simulink model "balancing_sim_model_induced_voltage"  (R2016a)
settings: Solver=ode4  StartTime=0.0  StopTime=Tfinal  FixedStep=Ts  RelTol=1e-3
values from neighbouring files (symbols this model uses):
  Cdc = 15e-6    (= 1.5e-05)    [balancing_sim_parameters.m]    (also in rectifier_sim_parameters.m; sixthharmonicstudies_another_sim_param.m)
  delta1 = acos(Ef1_avg/Vt1)    [balancing_sim_parameters.m]
  delta2 = acos(Ef2_avg/Vt2)    [balancing_sim_parameters.m]
  Ef1A = 80    [balancing_sim_parameters.m]
  Ef1A_ph = 0    [balancing_sim_parameters.m]
  Ef1B = Ef1A    (= 80)    [balancing_sim_parameters.m]
  Ef1B_ph = Ef1A_ph - 120    (= -120)    [balancing_sim_parameters.m]
  Ef1C = Ef1A    (= 80)    [balancing_sim_parameters.m]
  Ef1C_ph = Ef1A_ph + 120    (= 120)    [balancing_sim_parameters.m]
  Ef2A = 90    [balancing_sim_parameters.m]
  Ef2A_ph = 0    [balancing_sim_parameters.m]
  Ef2B = Ef2A    (= 90)    [balancing_sim_parameters.m]
  Ef2B_ph = Ef2A_ph - 120    (= -120)    [balancing_sim_parameters.m]
  Ef2C = Ef2A    (= 90)    [balancing_sim_parameters.m]
  Ef2C_ph = Ef2A_ph + 120    (= 120)    [balancing_sim_parameters.m]
  fout = 75    [balancing_sim_parameters.m]    (also in balancing_voltage_calc.m = 50; rectifier_sim_parameters.m = 50; sixthharmonicstudies_another_sim_param.m = 150)
  Ls = 10e-3    (= 0.01)    [balancing_sim_parameters.m]
  ma1 = 0.9    [balancing_sim_parameters.m]    (also in balancing_voltage_calc.m; rectifier_sim_parameters.m; sixthharmonicstudies_another_sim_param.m)
  ma2 = 0.9    [balancing_sim_parameters.m]    (also in balancing_voltage_calc.m)
  phase = [0 90 0 90]    [balancing_sim_parameters.m]    (also in rectifier_sim_parameters.m; sixthharmonicstudies_another_sim_param.m)
  Rin = 70    [balancing_sim_parameters.m]    (also in rectifier_sim_parameters.m = 10; sixthharmonicstudies_another_sim_param.m = 10)
  Ripth = 0.04    [balancing_sim_parameters.m]    (also in rectifier_sim_parameters.m = 0.18; sixthharmonicstudies_another_sim_param.m = 0.18)
  Rs = 1e-3    (= 0.001)    [balancing_sim_parameters.m]
  Ts = 1e-7    (= 1e-07)    [balancing_sim_parameters.m]    (also in rectifier_sim_parameters.m = 1e-06; sixthharmonicstudies_another_sim_param.m = 1e-06)
  Vin = Vdc + Rin*(Pout/Vdc)+3    (= 1061.51851852)    [balancing_sim_parameters.m]    (also in rectifier_sim_parameters.m = 366.296296296; sixthharmonicstudies_another_sim_param.m = 344.814814815)
  wout = 2*pi*fout    (= 471.238898038)    [balancing_sim_parameters.m]    (also in rectifier_sim_parameters.m = 314.159265359; sixthharmonicstudies_another_sim_param.m = 942.477796077)
undefined symbols (not defined in the file or in its folder): Lload, Rload
libraries: powerlib x47, powerlib_meascontrol x29, simulink x8
settings Model: SimulationMode=accelerator  Creator=ugurm  LastModifiedBy=mesutto
settings DataIOCC: LimitDataPoints=on  SaveFormat=Array
settings DebuggingCC: UnderspecifiedInitializationDetection=Classic  MergeDetectMultiDrivingBlocksExec=none  SolverPrmCheckMsg=warning  StateNameClashWarn=warning
settings HardwareCC: ProdBitPerPointer=32  ProdLargestAtomicFloat=None  ProdIntDivRoundTo=Undefined  ProdEndianess=Unspecified  ProdWordSize=32  ProdHWDeviceType=32-bit Generic
settings ModelReferenceCC: PropagateSignalLabelsOutOfModel=off
settings ConfigComp: CovModelRefEnable=Off

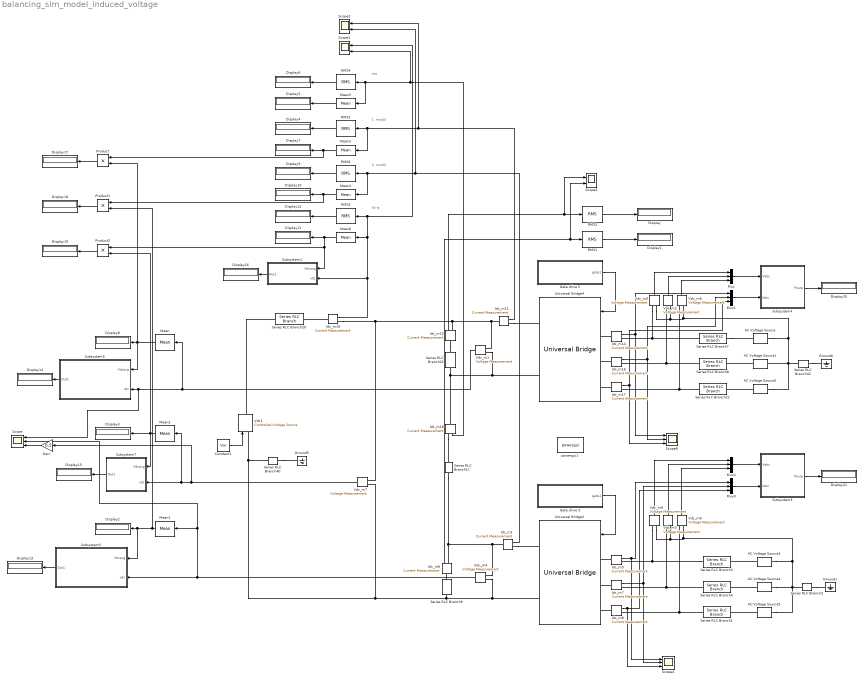
== system balancing_sim_model_induced_voltage ==
  note: 1. modül
  note: 2. modül
  note: ara
  note: Giriş
  AC Voltage Source : powerlib/Electrical Sources/AC Voltage Source  Amplitude=Ef1A*sqrt(2)  Phase=Ef1A_ph  Frequency=fout  SampleTime=0  Measurements=None  BusType=swing  Pref=10e3  Qref=0  Qmin=-inf  Qmax=+inf
  AC Voltage Source1 : powerlib/Electrical Sources/AC Voltage Source  Amplitude=Ef1B*sqrt(2)  Phase=Ef1B_ph  Frequency=fout  SampleTime=0  Measurements=None  BusType=swing  Pref=10e3  Qref=0  Qmin=-inf  Qmax=+inf
  AC Voltage Source2 : powerlib/Electrical Sources/AC Voltage Source  Amplitude=Ef1C*sqrt(2)  Phase=Ef1C_ph  Frequency=fout  SampleTime=0  Measurements=None  BusType=swing  Pref=10e3  Qref=0  Qmin=-inf  Qmax=+inf
  AC Voltage Source3 : powerlib/Electrical Sources/AC Voltage Source  Amplitude=Ef2A*sqrt(2)  Phase=Ef2A_ph  Frequency=fout  SampleTime=0  Measurements=None  BusType=swing  Pref=10e3  Qref=0  Qmin=-inf  Qmax=+inf
  AC Voltage Source4 : powerlib/Electrical Sources/AC Voltage Source  Amplitude=Ef2B*sqrt(2)  Phase=Ef2B_ph  Frequency=fout  SampleTime=0  Measurements=None  BusType=swing  Pref=10e3  Qref=0  Qmin=-inf  Qmax=+inf
  AC Voltage Source5 : powerlib/Electrical Sources/AC Voltage Source  Amplitude=Ef2C*sqrt(2)  Phase=Ef2C_ph  Frequency=fout  SampleTime=0  Measurements=None  BusType=swing  Pref=10e3  Qref=0  Qmin=-inf  Qmax=+inf
  Constant1 : Constant  Value=Vin
  Display{,1..21} (22 alike) : Display
  Gain : Gain  Gain=0.5
  Gate drive 3 : Subsystem
  Gate drive 5 : Subsystem
  Ground1 : powerlib/Elements/Ground  LConnTagsString=a
  Ground5 : powerlib/Elements/Ground  LConnTagsString=a
  Ground6 : powerlib/Elements/Ground  LConnTagsString=a
  Idc_m{1,5..8,11,14..19} (12 alike) : powerlib/Measurements/Current Measurement  PhasorSimulation=off  OutputType=Complex  PSBequivalent=0
  Mean{,1..6} (7 alike) : powerlib_meascontrol/Measurements/Mean  Freq=fout  Vinit=0  Ts=0
  Mux{,1..3} (4 alike) : Mux  Inputs=3
  Product : Product
  Product1 : Product
  Product2 : Product
  RMS{1..6} (6 alike) : powerlib_meascontrol/Measurements/RMS  TrueRMS=on  Freq=fout  RMSInit=0  Ts=0
  Scope : Scope  NumInputPorts=3
  Scope1 : Scope  NumInputPorts=2
  Scope2 : Scope  NumInputPorts=2
  Scope3 : Scope  NumInputPorts=2
  Scope4 : Scope  NumInputPorts=3
  Scope8 : Scope  NumInputPorts=3
  Series RLC Branch{1,3..4,7..8,22} (6 alike) : powerlib/Elements/Series RLC Branch  LConnTagsString=__new0  RConnTagsString=__new0  BranchType=RL  Resistance=Rs  Inductance=Ls  SetiL0=off  InitialCurrent=0  Capacitance=1e-6  Setx0=off  InitialVoltage=0  Measurements=None
  Series RLC Branch17 : powerlib/Elements/Series RLC Branch  LConnTagsString=__new0  RConnTagsString=__new0  BranchType=R  Resistance=1e-6  Inductance=Lload  SetiL0=off  InitialCurrent=0  Capacitance=1e-6  Setx0=off  InitialVoltage=0  Measurements=None
  Series RLC Branch2 : powerlib/Elements/Series RLC Branch  LConnTagsString=__new0  RConnTagsString=__new0  BranchType=R  Resistance=1e12  Inductance=Lload  SetiL0=off  InitialCurrent=0  Capacitance=1e-6  Setx0=off  InitialVoltage=0  Measurements=None
  Series RLC Branch20 : powerlib/Elements/Series RLC Branch  LConnTagsString=__new0  RConnTagsString=__new0  BranchType=R  Resistance=Rin  Inductance=1e-3  SetiL0=off  InitialCurrent=0  Capacitance=1e-6  Setx0=off  InitialVoltage=0  Measurements=None
  Series RLC Branch21 : powerlib/Elements/Series RLC Branch  LConnTagsString=__new0  RConnTagsString=__new0  BranchType=C  Resistance=Rload  Inductance=Lload  SetiL0=off  InitialCurrent=0  Capacitance=Cdc  Setx0=off  InitialVoltage=0  Measurements=None
  Series RLC Branch40 : powerlib/Elements/Series RLC Branch  LConnTagsString=__new0  RConnTagsString=__new0  BranchType=R  Resistance=1e12  Inductance=Lload  SetiL0=off  InitialCurrent=0  Capacitance=1e-6  Setx0=off  InitialVoltage=0  Measurements=None
  Series RLC Branch42 : powerlib/Elements/Series RLC Branch  LConnTagsString=__new0  RConnTagsString=__new0  BranchType=R  Resistance=1e12  Inductance=Lload  SetiL0=off  InitialCurrent=0  Capacitance=1e-6  Setx0=off  InitialVoltage=0  Measurements=None
  Series RLC Branch9 : powerlib/Elements/Series RLC Branch  LConnTagsString=__new0  RConnTagsString=__new0  BranchType=C  Resistance=Rload  Inductance=Lload  SetiL0=off  InitialCurrent=0  Capacitance=Cdc  Setx0=off  InitialVoltage=0  Measurements=None
  Subsystem1 : Subsystem
  Subsystem2 : Subsystem
  Subsystem3 : Subsystem
  Subsystem4 : Subsystem
  Subsystem5 : Subsystem
  Subsystem7 : Subsystem
  Universal Bridge3 : powerlib/Power Electronics/Universal Bridge  Arms=3  SnubberResistance=1e5  SnubberCapacitance=inf  Device=IGBT / Diodes  Ron=1e-6  Lon=0  ForwardVoltages="[  0  0  ]"  ForwardVoltage=0  GTOparameters=[ 10e-6 , 20e-6 ]  IGBTparameters=[0,0]  Measurements=None  Measurements_2=None  converterType=Rectifier
  Universal Bridge4 : powerlib/Power Electronics/Universal Bridge  Arms=3  SnubberResistance=1e5  SnubberCapacitance=inf  Device=IGBT / Diodes  Ron=1e-6  Lon=0  ForwardVoltages="[  0  0  ]"  ForwardVoltage=0  GTOparameters=[ 10e-6 , 20e-6 ]  IGBTparameters=[0,0]  Measurements=None  Measurements_2=None  converterType=Rectifier
  Vdc1 : powerlib/Electrical Sources/Controlled Voltage Source  Initialize=off  Source_Type=DC  Amplitude=200  Phase=0  Frequency=0  Measurements=None
  Vdc_m{1..9} (9 alike) : powerlib/Measurements/Voltage Measurement  PhasorSimulation=off  OutputType=Complex  PSBequivalent=0
  powergui1 : powerlib/powergui  Priority=1  SimulationMode=Discrete  SolverType=Tustin  SampleTime=Ts  frequency=60  SPID=off  DisableSnubberDevices=off  DisableRonSwitches=off  DisableVfSwitches=off  SwTol=0  DisplayEquations=off  Interpol=off  ExternalGateDelay=off  methode=off  Ts=0  FunctionMessages=off  echomessages=off  HookPort=off  EnableUseOfTLC=off  x0status=blocks  frequencyindice=0  Pbase=100e6  ErrMax=1e-4  Iterations=50  UnitsV=kV  UnitsW=MW  buscounter=0  RestoreLinks=warning  ResistiveCurrentMeasurement=off  Frange=[0:2:500]  Ylog=off  Xlog=on  ShowGrid=off  save=off  variable=ZData  structure=Vdc  ZoomFFT=off  StartTime=0.04  cycles=5  DisplayStyle=5  fundamental=50  FreqAxis=off  MaxFrequency=30000  frequencyindicesteady=1  RmsSteady=1  display=off
  wires:
  Gate drive 5/1(gate1) -> Universal Bridge4/1
  Idc_m14/1 -> Mux1/1, Scope8/1
  Constant1/1 -> Vdc1/1
  Idc_m15/1 -> RMS3/1, Scope3/1
  Vdc_m1/1 -> Mean/1, Scope/1, Subsystem5/2(vdc)
  Idc_m16/1 -> Mux1/2, Scope8/2
  Idc_m17/1 -> Scope8/3, Mux1/3
  RMS3/1 -> Display/1
  Mean/1 -> Product/2, Subsystem5/1(Vdcavg), Display8/1
  Gate drive 3/1(gate1) -> Universal Bridge3/1
  Mean1/1 -> Product1/2, Subsystem2/1(Vdcavg), Display2/1
  Mean2/1 -> Product2/2, Subsystem7/1(Vdcavg), Display3/1
  Vdc_m7/1 -> Gain/1, Subsystem7/2(vdc), Mean2/1
  RMS2/1 -> Display4/1
  Idc_m11/1 -> RMS2/1, Mean3/1, Scope2/1
  Idc_m18/1 -> Scope1/2, Mean5/1, RMS4/1
  Idc_m19/1 -> Subsystem1/2(vdc), Mean6/1, Scope1/1, RMS5/1
  Idc_m6/1 -> Scope3/2, RMS1/1
  RMS1/1 -> Display1/1
  Mean3/1 -> Product/1, Display7/1
  RMS6/1 -> Display9/1
  Mean4/1 -> Display10/1, Product1/1
  RMS4/1 -> Display6/1
  Mean5/1 -> Display5/1
  RMS5/1 -> Display12/1
  Mean6/1 -> Product2/1, Subsystem1/1(Vdcavg), Display11/1
  Idc_m1/1 -> Mean4/1, RMS6/1, Scope2/2
  Subsystem5/1(Out1) -> Display14/1
  Subsystem2/1(Out1) -> Display13/1
  Subsystem7/1(Out1) -> Display15/1
  Subsystem1/1(Out1) -> Display16/1
  Product/1 -> Display17/1
  Product1/1 -> Display18/1
  Vdc_m4/1 -> Scope/2, Mean1/1, Subsystem2/2(vdc)
  Product2/1 -> Display19/1
  Vdc_m5/1 -> Mux/1
  Vdc_m2/1 -> Mux/2
  Vdc_m6/1 -> Mux/3
  Mux/1 -> Subsystem4/1(Vabc)
  Mux1/1 -> Subsystem4/2(Iabc)
  Vdc_m8/1 -> Mux2/1
  Vdc_m3/1 -> Mux2/2
  Vdc_m9/1 -> Mux2/3
  Mux2/1 -> Subsystem3/1(Vabc)
  Mux3/1 -> Subsystem3/2(Iabc)
  Idc_m5/1 -> Scope4/1, Mux3/1
  Idc_m7/1 -> Scope4/2, Mux3/2
  Idc_m8/1 -> Scope4/3, Mux3/3
  Subsystem4/1(Poutp) -> Display20/1
  Subsystem3/1(Poutp) -> Display21/1
  Gain/1 -> Scope/3
  connections:
  Vdc_m5/LConn1 -- Series RLC Branch7/LConn1 -- Idc_m14/RConn1
  Idc_m18/LConn1 -- Vdc_m1/LConn2 -- Universal Bridge4/RConn2 -- Series RLC Branch21/RConn1
  Series RLC Branch42/RConn1 -- Ground6/LConn1
  Series RLC Branch40/RConn1 -- Ground5/LConn1
  Idc_m14/LConn1 -- Universal Bridge4/LConn1
  Idc_m15/LConn1 -- Series RLC Branch21/LConn1
  Vdc1/RConn1 -- Series RLC Branch20/LConn1
  Idc_m16/LConn1 -- Universal Bridge4/LConn2
  Idc_m17/LConn1 -- Universal Bridge4/LConn3
  Vdc_m6/LConn1 -- Series RLC Branch22/LConn1 -- Idc_m17/RConn1
  Vdc_m2/LConn1 -- Series RLC Branch8/LConn1 -- Idc_m16/RConn1
  Vdc_m8/LConn1 -- Series RLC Branch3/LConn1 -- Idc_m5/RConn1
  Series RLC Branch2/LConn1 -- AC Voltage Source4/LConn1 -- AC Voltage Source5/LConn1 -- AC Voltage Source3/LConn1 -- Vdc_m3/LConn2 -- Vdc_m8/LConn2 -- Vdc_m9/LConn2
  Vdc_m3/LConn1 -- Series RLC Branch4/LConn1 -- Idc_m7/RConn1
  Vdc_m9/LConn1 -- Series RLC Branch1/LConn1 -- Idc_m8/RConn1
  Idc_m8/LConn1 -- Universal Bridge3/LConn3
  Idc_m5/LConn1 -- Universal Bridge3/LConn1
  Idc_m7/LConn1 -- Universal Bridge3/LConn2
  Idc_m6/LConn1 -- Series RLC Branch9/LConn1
  Idc_m15/RConn1 -- Vdc_m1/LConn1 -- Idc_m11/LConn1 -- Vdc_m7/LConn1 -- Idc_m19/RConn1
  Series RLC Branch17/RConn1 -- Vdc_m4/LConn1 -- Idc_m1/LConn1 -- Idc_m6/RConn1
  Idc_m11/RConn1 -- Universal Bridge4/RConn1
  Idc_m18/RConn1 -- Series RLC Branch17/LConn1
  Idc_m19/LConn1 -- Series RLC Branch20/RConn1
  Vdc1/LConn1 -- Vdc_m4/LConn2 -- Universal Bridge3/RConn2 -- Series RLC Branch9/RConn1 -- Vdc_m7/LConn2 -- Series RLC Branch40/LConn1
  Idc_m1/RConn1 -- Universal Bridge3/RConn1
  Vdc_m5/LConn2 -- Series RLC Branch42/LConn1 -- AC Voltage Source2/LConn1 -- AC Voltage Source1/LConn1 -- AC Voltage Source/LConn1 -- Vdc_m6/LConn2 -- Vdc_m2/LConn2
  AC Voltage Source1/RConn1 -- Series RLC Branch8/RConn1
  Series RLC Branch7/RConn1 -- AC Voltage Source/RConn1
  AC Voltage Source2/RConn1 -- Series RLC Branch22/RConn1
  AC Voltage Source4/RConn1 -- Series RLC Branch4/RConn1
  AC Voltage Source3/RConn1 -- Series RLC Branch3/RConn1
  AC Voltage Source5/RConn1 -- Series RLC Branch1/RConn1
  Series RLC Branch2/RConn1 -- Ground1/LConn1

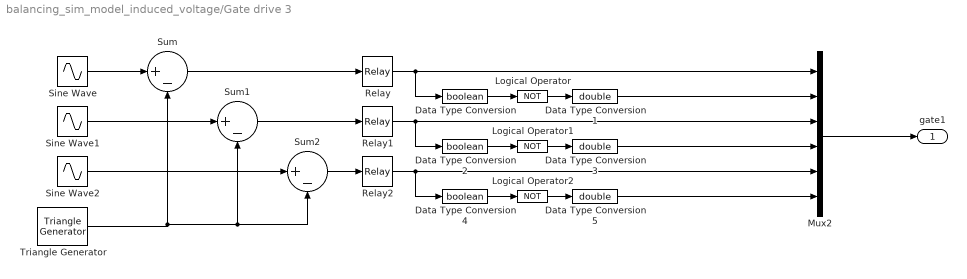
== system balancing_sim_model_induced_voltage/Gate drive 3 ==
  Data Type Conversion : DataTypeConversion  OutDataTypeStr=boolean
  Data Type Conversion1 : DataTypeConversion  OutDataTypeStr=double
  Data Type Conversion2 : DataTypeConversion  OutDataTypeStr=boolean
  Data Type Conversion3 : DataTypeConversion  OutDataTypeStr=double
  Data Type Conversion4 : DataTypeConversion  OutDataTypeStr=boolean
  Data Type Conversion5 : DataTypeConversion  OutDataTypeStr=double
  Logical Operator : Logic  Operator=NOT  AllPortsSameDT=off  OutDataTypeStr=boolean
  Logical Operator1 : Logic  Operator=NOT  AllPortsSameDT=off  OutDataTypeStr=boolean
  Logical Operator2 : Logic  Operator=NOT  AllPortsSameDT=off  OutDataTypeStr=boolean
  Mux2 : Mux  Inputs=6
  Relay : Relay
  Relay1 : Relay
  Relay2 : Relay
  Sine Wave : Sin  Amplitude=ma2  Frequency=wout  Phase=delta2  SampleTime=0
  Sine Wave1 : Sin  Amplitude=ma2  Frequency=wout  Phase=-2*pi/3+delta2  SampleTime=0
  Sine Wave2 : Sin  Amplitude=ma2  Frequency=wout  Phase=2*pi/3+delta2  SampleTime=0
  Sum : Sum  Inputs=|+-
  Sum1 : Sum  Inputs=|+-
  Sum2 : Sum  Inputs=|+-
  Triangle Generator : powerlib_meascontrol/Pulse & Signal Generators/Triangle Generator  Freq=fsw  Phase=phase(3)  Ts=Ts
  gate1 : Outport
  wires:
  Sine Wave/1 -> Sum/1
  Triangle Generator/1 -> Sum1/2, Sum2/2, Sum/2
  Sine Wave1/1 -> Sum1/1
  Sine Wave2/1 -> Sum2/1
  Sum/1 -> Relay/1
  Sum1/1 -> Relay1/1
  Sum2/1 -> Relay2/1
  Data Type Conversion/1 -> Logical Operator/1
  Relay/1 -> Data Type Conversion/1, Mux2/1
  Logical Operator/1 -> Data Type Conversion1/1
  Data Type Conversion1/1 -> Mux2/2
  Data Type Conversion2/1 -> Logical Operator1/1
  Relay1/1 -> Data Type Conversion2/1, Mux2/3
  Logical Operator1/1 -> Data Type Conversion3/1
  Data Type Conversion3/1 -> Mux2/4
  Data Type Conversion4/1 -> Logical Operator2/1
  Relay2/1 -> Data Type Conversion4/1, Mux2/5
  Logical Operator2/1 -> Data Type Conversion5/1
  Data Type Conversion5/1 -> Mux2/6
  Mux2/1 -> gate1/1

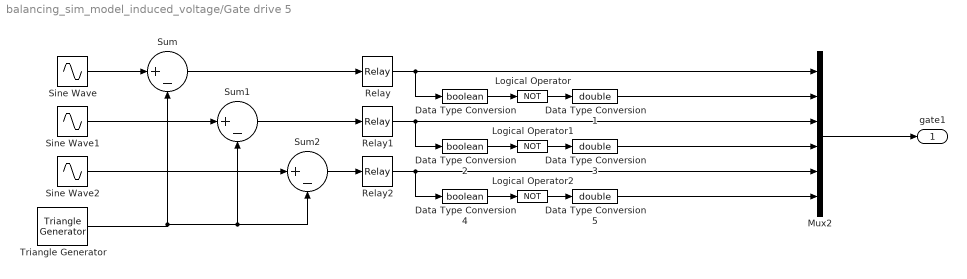
== system balancing_sim_model_induced_voltage/Gate drive 5 ==
  Data Type Conversion : DataTypeConversion  OutDataTypeStr=boolean
  Data Type Conversion1 : DataTypeConversion  OutDataTypeStr=double
  Data Type Conversion2 : DataTypeConversion  OutDataTypeStr=boolean
  Data Type Conversion3 : DataTypeConversion  OutDataTypeStr=double
  Data Type Conversion4 : DataTypeConversion  OutDataTypeStr=boolean
  Data Type Conversion5 : DataTypeConversion  OutDataTypeStr=double
  Logical Operator : Logic  Operator=NOT  AllPortsSameDT=off  OutDataTypeStr=boolean
  Logical Operator1 : Logic  Operator=NOT  AllPortsSameDT=off  OutDataTypeStr=boolean
  Logical Operator2 : Logic  Operator=NOT  AllPortsSameDT=off  OutDataTypeStr=boolean
  Mux2 : Mux  Inputs=6
  Relay : Relay
  Relay1 : Relay
  Relay2 : Relay
  Sine Wave : Sin  Amplitude=ma1  Frequency=wout  Phase=delta1  SampleTime=0
  Sine Wave1 : Sin  Amplitude=ma1  Frequency=wout  Phase=-2*pi/3+delta1  SampleTime=0
  Sine Wave2 : Sin  Amplitude=ma1  Frequency=wout  Phase=2*pi/3+delta1  SampleTime=0
  Sum : Sum  Inputs=|+-
  Sum1 : Sum  Inputs=|+-
  Sum2 : Sum  Inputs=|+-
  Triangle Generator : powerlib_meascontrol/Pulse & Signal Generators/Triangle Generator  Freq=fsw  Phase=phase(1)  Ts=Ts
  gate1 : Outport
  wires:
  Sine Wave/1 -> Sum/1
  Triangle Generator/1 -> Sum1/2, Sum2/2, Sum/2
  Sine Wave1/1 -> Sum1/1
  Sine Wave2/1 -> Sum2/1
  Sum/1 -> Relay/1
  Sum1/1 -> Relay1/1
  Sum2/1 -> Relay2/1
  Data Type Conversion/1 -> Logical Operator/1
  Relay/1 -> Data Type Conversion/1, Mux2/1
  Logical Operator/1 -> Data Type Conversion1/1
  Data Type Conversion1/1 -> Mux2/2
  Data Type Conversion2/1 -> Logical Operator1/1
  Relay1/1 -> Data Type Conversion2/1, Mux2/3
  Logical Operator1/1 -> Data Type Conversion3/1
  Data Type Conversion3/1 -> Mux2/4
  Data Type Conversion4/1 -> Logical Operator2/1
  Relay2/1 -> Data Type Conversion4/1, Mux2/5
  Logical Operator2/1 -> Data Type Conversion5/1
  Data Type Conversion5/1 -> Mux2/6
  Mux2/1 -> gate1/1

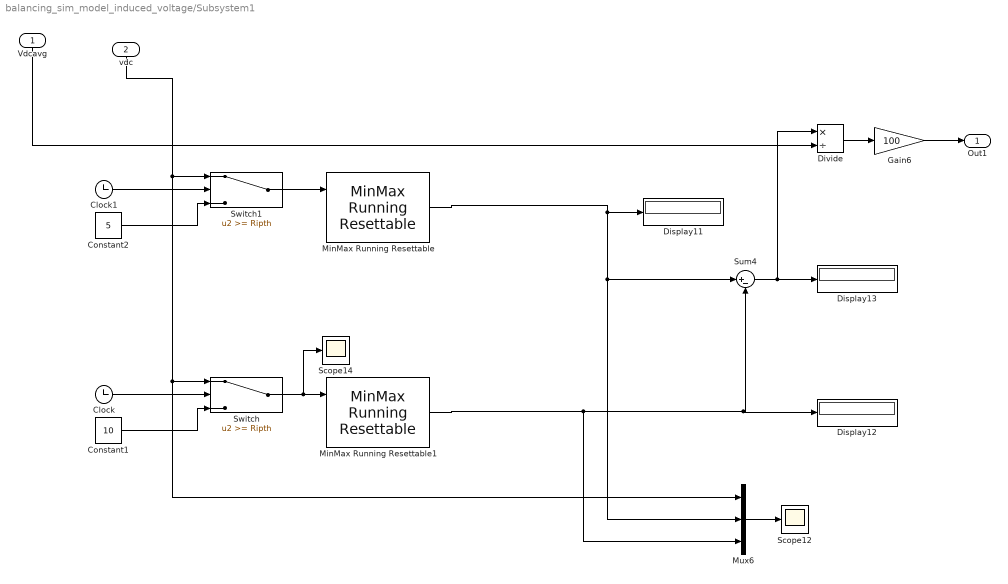
== system balancing_sim_model_induced_voltage/Subsystem1 ==
  Vdcavg : Inport
  vdc : Inport  Port=2
  Clock : Clock
  Clock1 : Clock
  Constant1 : Constant  Value=10  SampleTime=Ts
  Constant2 : Constant  Value=5  SampleTime=Ts
  Display11 : Display
  Display12 : Display
  Display13 : Display
  Divide : Product  Inputs=*/
  Gain6 : Gain  Gain=100
  MinMax Running Resettable : simulink/Math Operations/MinMax Running Resettable  Function=max  vinit=0.0
  MinMax Running Resettable1 : simulink/Math Operations/MinMax Running Resettable  Function=min  vinit=700
  Mux6 : Mux  Inputs=3
  Scope12 : Scope
  Scope14 : Scope
  Sum4 : Sum  Inputs=|+-
  Switch : Switch  Threshold=Ripth
  Switch1 : Switch  Threshold=Ripth
  Out1 : Outport
  wires:
  MinMax Running Resettable/1 -> Display11/1, Mux6/2, Sum4/1
  Clock/1 -> Switch/2
  Gain6/1 -> Out1/1
  Constant1/1 -> Switch/3
  MinMax Running Resettable1/1 -> Mux6/3, Display12/1, Sum4/2
  Switch/1 -> Scope14/1, MinMax Running Resettable1/1
  Sum4/1 -> Divide/1, Display13/1
  Divide/1 -> Gain6/1
  Mux6/1 -> Scope12/1
  Vdcavg/1 -> Divide/2
  vdc/1 -> Switch1/1, Mux6/1, Switch/1
  Switch1/1 -> MinMax Running Resettable/1
  Clock1/1 -> Switch1/2
  Constant2/1 -> Switch1/3

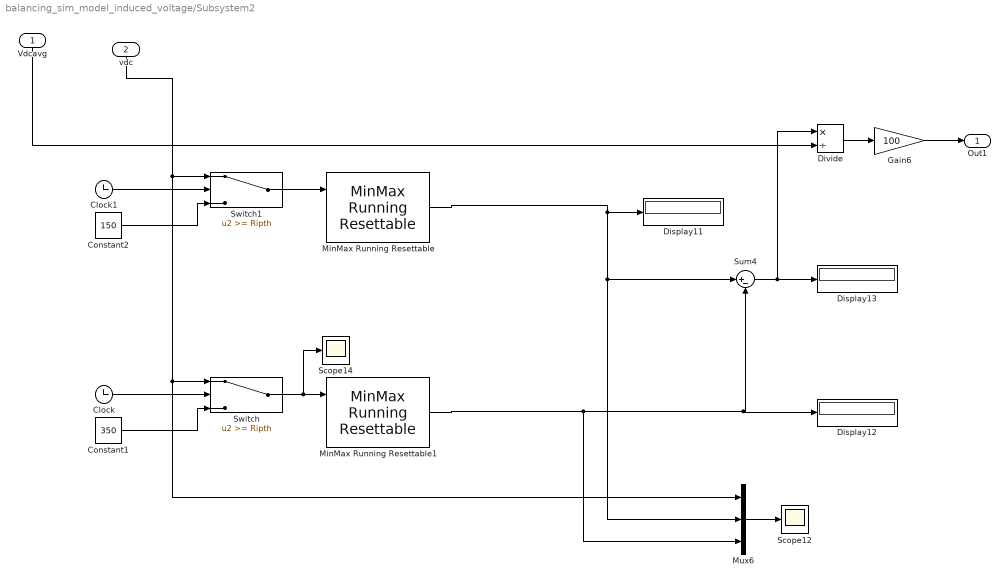
== system balancing_sim_model_induced_voltage/Subsystem2 ==
  Vdcavg : Inport
  vdc : Inport  Port=2
  Clock : Clock
  Clock1 : Clock
  Constant1 : Constant  Value=350  SampleTime=Ts
  Constant2 : Constant  Value=150  SampleTime=Ts
  Display11 : Display
  Display12 : Display
  Display13 : Display
  Divide : Product  Inputs=*/
  Gain6 : Gain  Gain=100
  MinMax Running Resettable : simulink/Math Operations/MinMax Running Resettable  Function=max  vinit=0.0
  MinMax Running Resettable1 : simulink/Math Operations/MinMax Running Resettable  Function=min  vinit=700
  Mux6 : Mux  Inputs=3
  Scope12 : Scope
  Scope14 : Scope
  Sum4 : Sum  Inputs=|+-
  Switch : Switch  Threshold=Ripth
  Switch1 : Switch  Threshold=Ripth
  Out1 : Outport
  wires:
  MinMax Running Resettable/1 -> Display11/1, Mux6/2, Sum4/1
  Clock/1 -> Switch/2
  Gain6/1 -> Out1/1
  Constant1/1 -> Switch/3
  MinMax Running Resettable1/1 -> Mux6/3, Display12/1, Sum4/2
  Switch/1 -> Scope14/1, MinMax Running Resettable1/1
  Sum4/1 -> Divide/1, Display13/1
  Divide/1 -> Gain6/1
  Mux6/1 -> Scope12/1
  Vdcavg/1 -> Divide/2
  vdc/1 -> Switch1/1, Mux6/1, Switch/1
  Switch1/1 -> MinMax Running Resettable/1
  Clock1/1 -> Switch1/2
  Constant2/1 -> Switch1/3

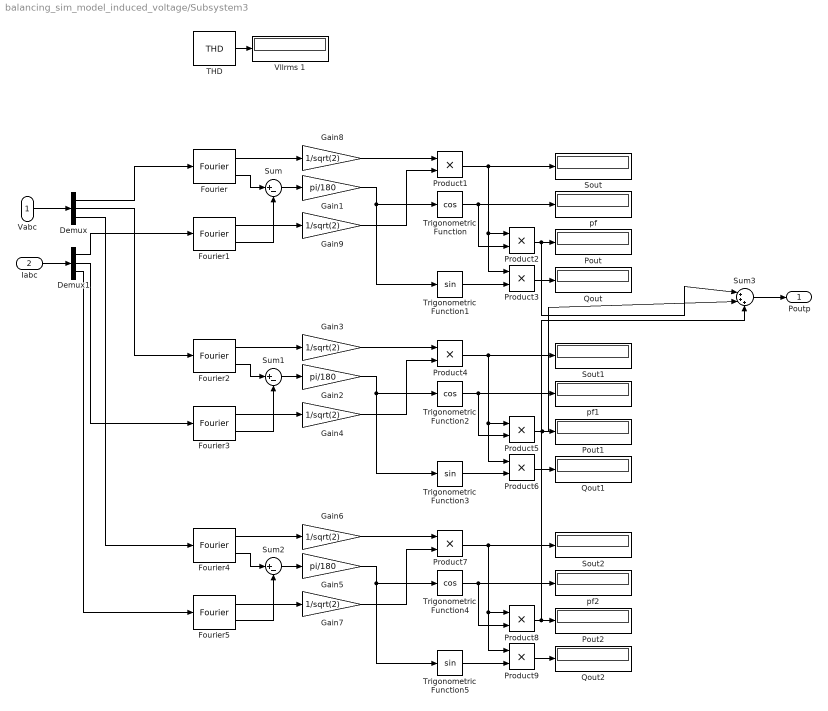
== system balancing_sim_model_induced_voltage/Subsystem3 ==
  Vabc : Inport
  Iabc : Inport  Port=2
  Demux : Demux  Outputs=3
  Demux1 : Demux  Outputs=3
  Fourier{,1..5} (6 alike) : powerlib_meascontrol/Measurements/Fourier  Freq=fout  n=1  InInit=[0, 0]  Ts=Ts
  Gain1 : Gain  Gain=pi/180
  Gain2 : Gain  Gain=pi/180
  Gain{3..4,6..9} (6 alike) : Gain  Gain=1/sqrt(2)
  Gain5 : Gain  Gain=pi/180
  Pout : Display
  Pout1 : Display
  Pout2 : Display
  Product{1..9} (9 alike) : Product
  Qout : Display
  Qout1 : Display
  Qout2 : Display
  Sout : Display
      settings: Format=short_e
  Sout1 : Display
      settings: Format=short_e
  Sout2 : Display
      settings: Format=short_e
  Sum : Sum  Inputs=|+-
  Sum1 : Sum  Inputs=|+-
  Sum2 : Sum  Inputs=|+-
  Sum3 : Sum  Inputs=|+++
  THD : powerlib_meascontrol/Measurements/THD  Freq=fout  Ts=0
  Trigonometric Function : Trigonometry  Operator=cos
  Trigonometric Function1 : Trigonometry
  Trigonometric Function2 : Trigonometry  Operator=cos
  Trigonometric Function3 : Trigonometry
  Trigonometric Function4 : Trigonometry  Operator=cos
  Trigonometric Function5 : Trigonometry
  Vllrms 1 : Display
  pf : Display
  pf1 : Display
  pf2 : Display
  Poutp : Outport
  wires:
  Gain8/1 -> Product1/1
  Gain9/1 -> Product1/2
  Fourier1/1 -> Gain9/1
  Fourier/1 -> Gain8/1
  Product1/1 -> Product3/1, Product2/1, Sout/1
  Sum/1 -> Gain1/1
  Trigonometric Function/1 -> Product2/2, pf/1
  Gain1/1 -> Trigonometric Function1/1, Trigonometric Function/1
  Product2/1 -> Sum3/1, Pout/1
  THD/1 -> Vllrms 1/1
  Vabc/1 -> Demux/1
  Iabc/1 -> Demux1/1
  Fourier/2 -> Sum/1
  Fourier1/2 -> Sum/2
  Trigonometric Function1/1 -> Product3/2
  Product3/1 -> Qout/1
  Gain3/1 -> Product4/1
  Gain4/1 -> Product4/2
  Fourier3/1 -> Gain4/1
  Fourier2/1 -> Gain3/1
  Product4/1 -> Product6/1, Product5/1, Sout1/1
  Sum1/1 -> Gain2/1
  Trigonometric Function2/1 -> Product5/2, pf1/1
  Gain2/1 -> Trigonometric Function3/1, Trigonometric Function2/1
  Product5/1 -> Sum3/2, Pout1/1
  Fourier2/2 -> Sum1/1
  Fourier3/2 -> Sum1/2
  Trigonometric Function3/1 -> Product6/2
  Product6/1 -> Qout1/1
  Gain6/1 -> Product7/1
  Gain7/1 -> Product7/2
  Fourier5/1 -> Gain7/1
  Fourier4/1 -> Gain6/1
  Product7/1 -> Product9/1, Product8/1, Sout2/1
  Sum2/1 -> Gain5/1
  Trigonometric Function4/1 -> Product8/2, pf2/1
  Gain5/1 -> Trigonometric Function5/1, Trigonometric Function4/1
  Fourier4/2 -> Sum2/1
  Fourier5/2 -> Sum2/2
  Trigonometric Function5/1 -> Product9/2
  Product9/1 -> Qout2/1
  Product8/1 -> Sum3/3, Pout2/1
  Sum3/1 -> Poutp/1
  Demux/1 -> Fourier/1
  Demux/2 -> Fourier2/1
  Demux/3 -> Fourier4/1
  Demux1/1 -> Fourier1/1
  Demux1/2 -> Fourier3/1
  Demux1/3 -> Fourier5/1

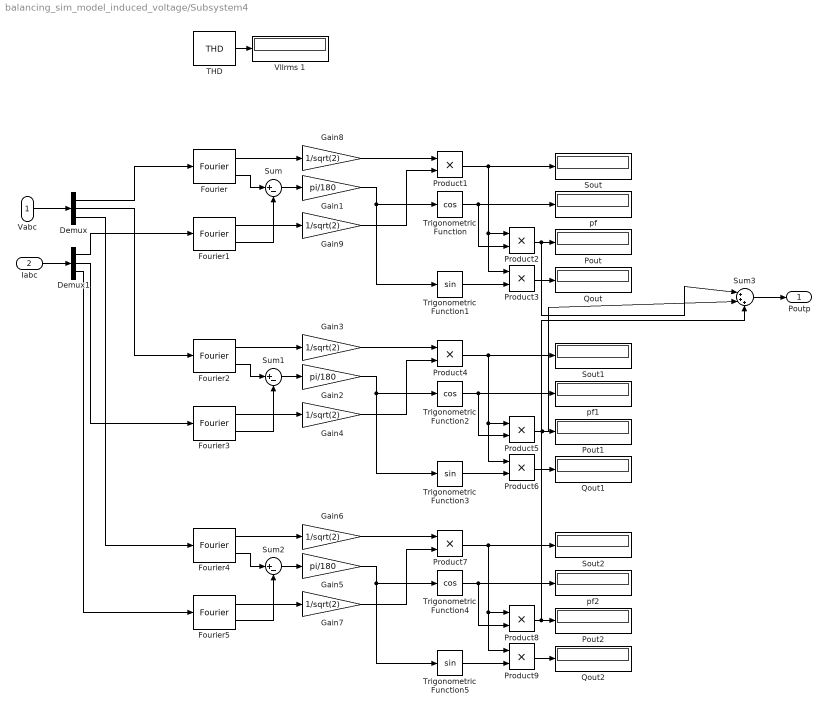
== system balancing_sim_model_induced_voltage/Subsystem4 ==
  Vabc : Inport
  Iabc : Inport  Port=2
  Demux : Demux  Outputs=3
  Demux1 : Demux  Outputs=3
  Fourier{,1..5} (6 alike) : powerlib_meascontrol/Measurements/Fourier  Freq=fout  n=1  InInit=[0, 0]  Ts=Ts
  Gain1 : Gain  Gain=pi/180
  Gain2 : Gain  Gain=pi/180
  Gain{3..4,6..9} (6 alike) : Gain  Gain=1/sqrt(2)
  Gain5 : Gain  Gain=pi/180
  Pout : Display
  Pout1 : Display
  Pout2 : Display
  Product{1..9} (9 alike) : Product
  Qout : Display
  Qout1 : Display
  Qout2 : Display
  Sout : Display
      settings: Format=short_e
  Sout1 : Display
      settings: Format=short_e
  Sout2 : Display
      settings: Format=short_e
  Sum : Sum  Inputs=|+-
  Sum1 : Sum  Inputs=|+-
  Sum2 : Sum  Inputs=|+-
  Sum3 : Sum  Inputs=|+++
  THD : powerlib_meascontrol/Measurements/THD  Freq=fout  Ts=0
  Trigonometric Function : Trigonometry  Operator=cos
  Trigonometric Function1 : Trigonometry
  Trigonometric Function2 : Trigonometry  Operator=cos
  Trigonometric Function3 : Trigonometry
  Trigonometric Function4 : Trigonometry  Operator=cos
  Trigonometric Function5 : Trigonometry
  Vllrms 1 : Display
  pf : Display
  pf1 : Display
  pf2 : Display
  Poutp : Outport
  wires:
  Gain8/1 -> Product1/1
  Gain9/1 -> Product1/2
  Fourier1/1 -> Gain9/1
  Fourier/1 -> Gain8/1
  Product1/1 -> Product3/1, Product2/1, Sout/1
  Sum/1 -> Gain1/1
  Trigonometric Function/1 -> Product2/2, pf/1
  Gain1/1 -> Trigonometric Function1/1, Trigonometric Function/1
  Product2/1 -> Sum3/1, Pout/1
  THD/1 -> Vllrms 1/1
  Vabc/1 -> Demux/1
  Iabc/1 -> Demux1/1
  Fourier/2 -> Sum/1
  Fourier1/2 -> Sum/2
  Trigonometric Function1/1 -> Product3/2
  Product3/1 -> Qout/1
  Gain3/1 -> Product4/1
  Gain4/1 -> Product4/2
  Fourier3/1 -> Gain4/1
  Fourier2/1 -> Gain3/1
  Product4/1 -> Product6/1, Product5/1, Sout1/1
  Sum1/1 -> Gain2/1
  Trigonometric Function2/1 -> Product5/2, pf1/1
  Gain2/1 -> Trigonometric Function3/1, Trigonometric Function2/1
  Product5/1 -> Sum3/2, Pout1/1
  Fourier2/2 -> Sum1/1
  Fourier3/2 -> Sum1/2
  Trigonometric Function3/1 -> Product6/2
  Product6/1 -> Qout1/1
  Gain6/1 -> Product7/1
  Gain7/1 -> Product7/2
  Fourier5/1 -> Gain7/1
  Fourier4/1 -> Gain6/1
  Product7/1 -> Product9/1, Product8/1, Sout2/1
  Sum2/1 -> Gain5/1
  Trigonometric Function4/1 -> Product8/2, pf2/1
  Gain5/1 -> Trigonometric Function5/1, Trigonometric Function4/1
  Fourier4/2 -> Sum2/1
  Fourier5/2 -> Sum2/2
  Trigonometric Function5/1 -> Product9/2
  Product9/1 -> Qout2/1
  Product8/1 -> Sum3/3, Pout2/1
  Sum3/1 -> Poutp/1
  Demux/1 -> Fourier/1
  Demux/2 -> Fourier2/1
  Demux/3 -> Fourier4/1
  Demux1/1 -> Fourier1/1
  Demux1/2 -> Fourier3/1
  Demux1/3 -> Fourier5/1

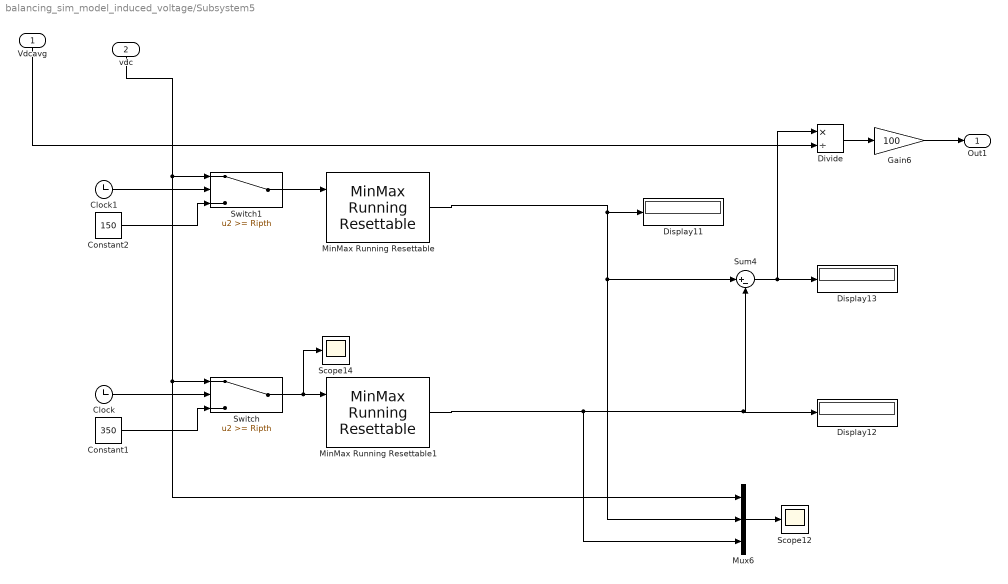
== system balancing_sim_model_induced_voltage/Subsystem5 ==
  Vdcavg : Inport
  vdc : Inport  Port=2
  Clock : Clock
  Clock1 : Clock
  Constant1 : Constant  Value=350  SampleTime=Ts
  Constant2 : Constant  Value=150  SampleTime=Ts
  Display11 : Display
  Display12 : Display
  Display13 : Display
  Divide : Product  Inputs=*/
  Gain6 : Gain  Gain=100
  MinMax Running Resettable : simulink/Math Operations/MinMax Running Resettable  Function=max  vinit=0.0
  MinMax Running Resettable1 : simulink/Math Operations/MinMax Running Resettable  Function=min  vinit=700
  Mux6 : Mux  Inputs=3
  Scope12 : Scope
  Scope14 : Scope
  Sum4 : Sum  Inputs=|+-
  Switch : Switch  Threshold=Ripth
  Switch1 : Switch  Threshold=Ripth
  Out1 : Outport
  wires:
  MinMax Running Resettable/1 -> Display11/1, Mux6/2, Sum4/1
  Clock/1 -> Switch/2
  Gain6/1 -> Out1/1
  Constant1/1 -> Switch/3
  MinMax Running Resettable1/1 -> Mux6/3, Display12/1, Sum4/2
  Switch/1 -> Scope14/1, MinMax Running Resettable1/1
  Sum4/1 -> Divide/1, Display13/1
  Divide/1 -> Gain6/1
  Mux6/1 -> Scope12/1
  Vdcavg/1 -> Divide/2
  vdc/1 -> Switch1/1, Mux6/1, Switch/1
  Switch1/1 -> MinMax Running Resettable/1
  Clock1/1 -> Switch1/2
  Constant2/1 -> Switch1/3

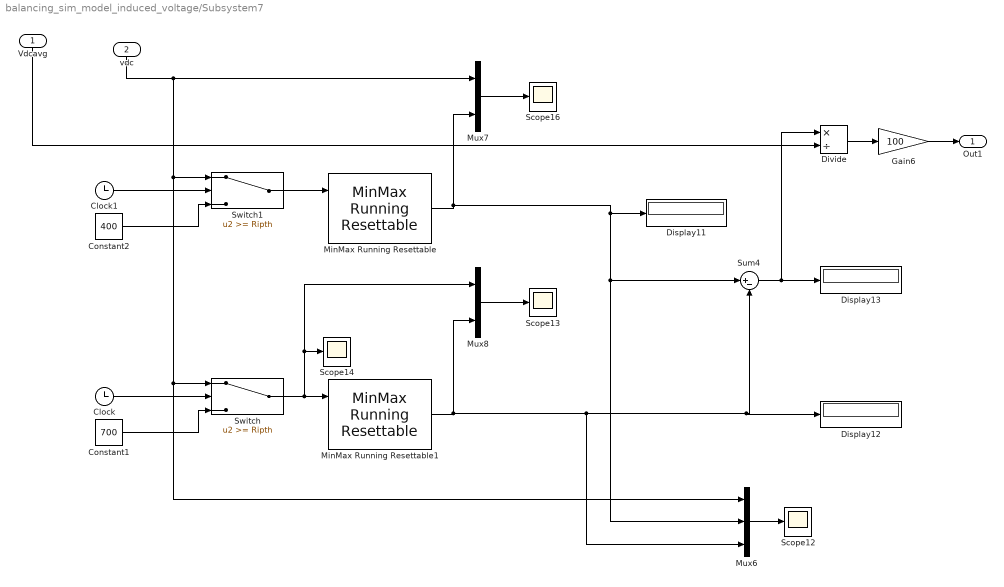
== system balancing_sim_model_induced_voltage/Subsystem7 ==
  Vdcavg : Inport
  vdc : Inport  Port=2
  Clock : Clock
  Clock1 : Clock
  Constant1 : Constant  Value=700  SampleTime=Ts
  Constant2 : Constant  Value=400  SampleTime=Ts
  Display11 : Display
  Display12 : Display
  Display13 : Display
  Divide : Product  Inputs=*/
  Gain6 : Gain  Gain=100
  MinMax Running Resettable : simulink/Math Operations/MinMax Running Resettable  Function=max  vinit=0.0
  MinMax Running Resettable1 : simulink/Math Operations/MinMax Running Resettable  Function=min  vinit=700
  Mux6 : Mux  Inputs=3
  Mux7 : Mux  Inputs=2
  Mux8 : Mux  Inputs=2
  Scope{12..14,16} (4 alike) : Scope
  Sum4 : Sum  Inputs=|+-
  Switch : Switch  Threshold=Ripth
  Switch1 : Switch  Threshold=Ripth
  Out1 : Outport
  wires:
  MinMax Running Resettable/1 -> Display11/1, Mux6/2, Sum4/1, Mux7/2
  Clock/1 -> Switch/2
  Mux8/1 -> Scope13/1
  Gain6/1 -> Out1/1
  Constant1/1 -> Switch/3
  MinMax Running Resettable1/1 -> Mux6/3, Display12/1, Sum4/2, Mux8/2
  Mux7/1 -> Scope16/1
  Switch/1 -> Mux8/1, Scope14/1, MinMax Running Resettable1/1
  Sum4/1 -> Divide/1, Display13/1
  Divide/1 -> Gain6/1
  Mux6/1 -> Scope12/1
  Vdcavg/1 -> Divide/2
  vdc/1 -> Mux7/1, Switch1/1, Mux6/1, Switch/1
  Switch1/1 -> MinMax Running Resettable/1
  Clock1/1 -> Switch1/2
  Constant2/1 -> Switch1/3
